simulink model "ploop_test"  (R2015a)
settings: Solver=ode15s  StartTime=0.0  StopTime=1  RelTol=1e-3
undefined symbols (not defined in the file): G
libraries: roblocks x2
settings Model: CovSFcnEnable=off  Creator=pic  LastModifiedBy=corkep
settings DataIOCC: LimitDataPoints=off  SignalLoggingSaveFormat=ModelDataLogs  ReturnWorkspaceOutputs=on  TimeSaveName=t  OutputSaveName=y  OutputOption=SpecifiedOutputTimes  OutputTimes=[0:0.001:1]'
settings OptimizationCC: ExpressionDepthLimit=2147483647
settings DebuggingCC: UnderspecifiedInitializationDetection=Classic  MergeDetectMultiDrivingBlocksExec=none  SolverPrmCheckMsg=warning  StateNameClashWarn=warning
settings GRTTargetCC: CombineOutputUpdateFcns=off  GRTInterface=on

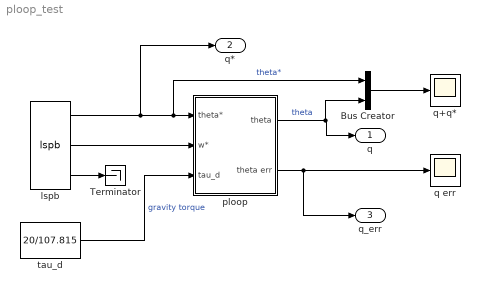
== system ploop_test ==
  Bus Creator : BusCreator  Inputs=2
  Terminator : Terminator
  lspb : roblocks/Toolbox/lspb  q0=0  qf=1  tmax=1
  ploop : Subsystem
  q err : Scope
      settings: TimeRange=1  LimitDataPoints=on  MaxDataPoints=5000  SaveToWorkspace=off  SaveName=ScopeData  YMin=-0.0051  YMax=0.04588  SampleTime=-1
  "q+q* " : Scope
      settings: TimeRange=auto  ShowLegends=on  LimitDataPoints=on  MaxDataPoints=5000  SaveToWorkspace=off  YMin=-0.12554  YMax=1.12506  SampleTime=-1
  tau_d : Constant  Value=20/107.815
  q : Outport
  q* : Outport  Port=2
  q_err : Outport  Port=3
  wires:
  ploop/1(theta) -> Bus Creator/2, q/1  "theta"
  ploop/2(theta err) -> q_err/1, q err/1
  lspb/1 -> q*/1, Bus Creator/1, ploop/1(theta*)  "theta*"
  tau_d/1 -> ploop/3(tau_d)  "gravity torque"
  lspb/3 -> Terminator/1
  lspb/2 -> ploop/2(w*)
  Bus Creator/1 -> "q+q* "/1

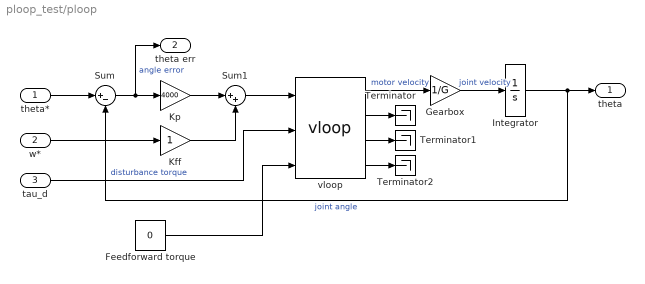
== system ploop_test/ploop ==
  theta* : Inport
  w* : Inport  Port=2
  tau_d : Inport  Port=3
  Feedforward torque : Constant  Value=0
  Gearbox : Gain  Gain=1/G
  Integrator : Integrator
  Kff : Gain
  Kp : Gain  Gain=4000
  Sum : Sum  Inputs=|+-
  Sum1 : Sum  Inputs=|++
  Terminator : Terminator
  Terminator1 : Terminator
  Terminator2 : Terminator
  vloop : roblocks/Arm/vloop  J=372e-6  B=817e-6  Km=0.228  tau_max=0.9  Kv=1  Ki=0  T=0.001
  theta : Outport
  theta err : Outport  Port=2
  wires:
  Sum/1 -> Kp/1, theta err/1  "angle error"
  Integrator/1 -> theta/1, Sum/2  "joint angle"
  theta*/1 -> Sum/1
  Kp/1 -> Sum1/1
  Sum1/1 -> vloop/1
  w*/1 -> Kff/1
  Kff/1 -> Sum1/2
  vloop/2 -> Terminator/1
  vloop/3 -> Terminator1/1
  vloop/4 -> Terminator2/1
  vloop/1 -> Gearbox/1  "motor velocity"
  tau_d/1 -> vloop/2  "disturbance torque"
  Feedforward torque/1 -> vloop/3
  Gearbox/1 -> Integrator/1  "joint velocity"
